simulink model "meat_1024pt_lwip_led"  (Simulink 6.2)
settings: Solver=ode45  StartTime=0.0  StopTime=20000  RelTol=1e-3
undefined symbols (not defined in the file): bit_rev, iBOB, pfb_coeff_gen_calc
libraries: xbsIndex_r3 x1078, casper_library x97, xps_library x30
(part 8 of 8)

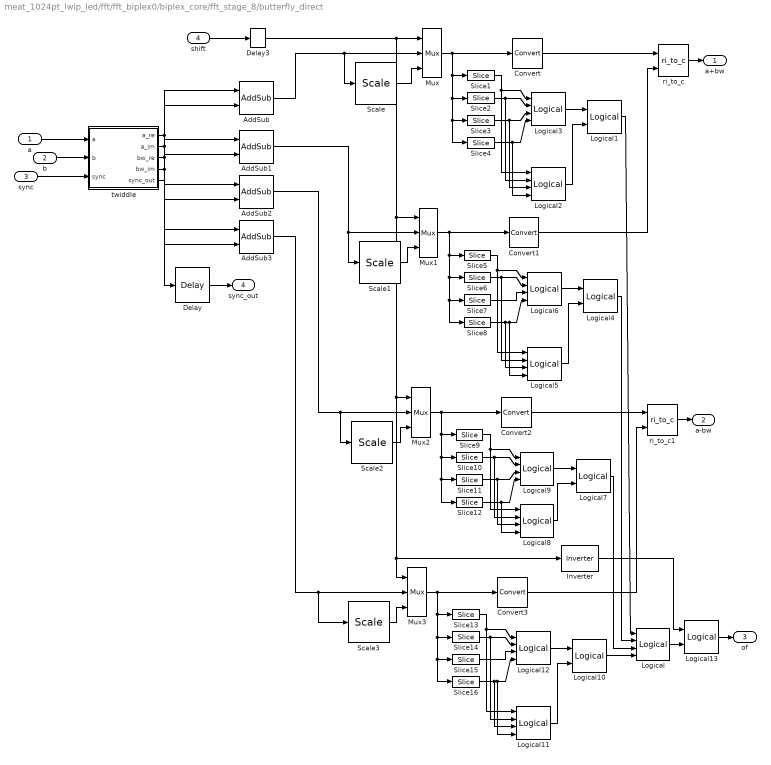
== system meat_1024pt_lwip_led/fft/fft_biplex0/biplex_core/fft_stage_8/butterfly_direct ==
  a : Inport  Port=1  LatchInput=off
  b : Inport  Port=2  LatchInput=off
  sync : Inport  Port=3  LatchInput=off
  shift : Inport  Port=4  LatchInput=off
  AddSub : xbsIndex_r3/AddSub  mode=Addition  precision=Full  arith_type=Unsigned  n_bits=8  bin_pt=2  quantization=Truncate  overflow=Wrap  latency=add_latency  explicit_period=off  period=1  use_carryin=off  use_carryout=off  en=off  dbl_ovrd=off  show_param=on  use_core=on  pipeline=on  use_rpm=on  gen_core=on
      settings: xl_area=[0, 0, 0, 0, 0, 0, 0]
  AddSub1 : xbsIndex_r3/AddSub  mode=Addition  precision=Full  arith_type=Unsigned  n_bits=8  bin_pt=2  quantization=Truncate  overflow=Wrap  latency=add_latency  explicit_period=off  period=1  use_carryin=off  use_carryout=off  en=off  dbl_ovrd=off  show_param=on  use_core=on  pipeline=on  use_rpm=on  gen_core=on
      settings: xl_area=[0, 0, 0, 0, 0, 0, 0]
  AddSub2 : xbsIndex_r3/AddSub  mode=Subtraction  precision=Full  arith_type=Unsigned  n_bits=8  bin_pt=2  quantization=Truncate  overflow=Wrap  latency=add_latency  explicit_period=off  period=1  use_carryin=off  use_carryout=off  en=off  dbl_ovrd=off  show_param=on  use_core=on  pipeline=on  use_rpm=on  gen_core=on
      settings: xl_area=[0, 0, 0, 0, 0, 0, 0]
  AddSub3 : xbsIndex_r3/AddSub  mode=Subtraction  precision=Full  arith_type=Unsigned  n_bits=8  bin_pt=2  quantization=Truncate  overflow=Wrap  latency=add_latency  explicit_period=off  period=1  use_carryin=off  use_carryout=off  en=off  dbl_ovrd=off  show_param=on  use_core=on  pipeline=on  use_rpm=on  gen_core=on
      settings: xl_area=[0, 0, 0, 0, 0, 0, 0]
  Convert{,1..3} (4 alike) : xbsIndex_r3/Convert  arith_type="Signed  (2's comp)"  n_bits=BitWidth  bin_pt=BitWidth-1  quantization=Truncate  overflow=Wrap  latency=add_latency  explicit_period=off  period=1  dbl_ovrd=off  show_param=off  inserted_by_tool=off  pipeline=off
      settings: xl_area=[0, 0, 0, 0, 0, 0, 0]
  Delay : xbsIndex_r3/Delay  latency=2 * add_latency + 1  reg_retiming=off  explicit_period=off  period=1  en=off  accept_only_valid=off  init_zero=on  dbl_ovrd=off  show_param=off
      settings: xl_area=[0, 0, 0, 0, 0, 0, 0]
  Delay3 : xbsIndex_r3/Delay  latency=1  reg_retiming=off  explicit_period=off  period=1  en=off  accept_only_valid=off  init_zero=on  dbl_ovrd=off  show_param=off
      settings: xl_area=[0, 0, 0, 0, 0, 0, 0]
  Inverter : xbsIndex_r3/Inverter  latency=0  explicit_period=off  period=1  en=off  dbl_ovrd=off  show_param=off
      settings: xl_area=[0, 0, 0, 0, 0, 0, 0]
  Logical : xbsIndex_r3/Logical  logical_function=OR  inputs=4  precision=Full  arith_type=Unsigned  n_bits=8  bin_pt=2  align_bp=on  latency=1  explicit_period=off  period=1  en=off  dbl_ovrd=off  show_param=off
      settings: xl_area=[0, 0, 0, 0, 0, 0, 0]
  Logical{1,4,7,10} (4 alike) : xbsIndex_r3/Logical  logical_function=OR  inputs=2  precision=Full  arith_type=Unsigned  n_bits=8  bin_pt=2  align_bp=off  latency=1  explicit_period=off  period=1  en=off  dbl_ovrd=off  show_param=off
      settings: xl_area=[0, 0, 0, 0, 0, 0, 0]
  Logical{2,5,8,11} (4 alike) : xbsIndex_r3/Logical  logical_function=NOR  inputs=4  precision=Full  arith_type=Unsigned  n_bits=8  bin_pt=2  align_bp=off  latency=1  explicit_period=off  period=1  en=off  dbl_ovrd=off  show_param=off
      settings: xl_area=[0, 0, 0, 0, 0, 0, 0]
  Logical{3,6,9,12} (4 alike) : xbsIndex_r3/Logical  logical_function=AND  inputs=4  precision=Full  arith_type=Unsigned  n_bits=8  bin_pt=2  align_bp=off  latency=1  explicit_period=off  period=1  en=off  dbl_ovrd=off  show_param=off
      settings: xl_area=[0, 0, 0, 0, 0, 0, 0]
  Logical13 : xbsIndex_r3/Logical  logical_function=AND  inputs=2  precision=Full  arith_type=Unsigned  n_bits=8  bin_pt=2  align_bp=off  latency=1  explicit_period=off  period=1  en=off  dbl_ovrd=off  show_param=off
      settings: xl_area=[0, 0, 0, 0, 0, 0, 0]
  Mux{,1..3} (4 alike) : xbsIndex_r3/Mux  inputs=2  precision=Full  arith_type="Signed  (2's comp)"  n_bits=8  bin_pt=2  quantization=Truncate  overflow=Wrap  latency=1  explicit_period=off  period=1  en=off  dbl_ovrd=off  show_param=off  mux_type=off  use_rpm=off  gen_core=off
      settings: xl_area=[0, 0, 0, 0, 0, 0, 0]
  Scale{,1..3} (4 alike) : xbsIndex_r3/Scale  scale_factor=-1  explicit_period=off  period=1  dbl_ovrd=off
  Slice{1,5,9,13} (4 alike) : xbsIndex_r3/Slice  mode=Upper Bit Location + Width  nbits=1  bit1=0  base1=MSB of Input  bit0=0  base0=LSB of Input  boolean_output=on  explicit_period=off  period=1  dbl_ovrd=off
  Slice{2,6,10,14} (4 alike) : xbsIndex_r3/Slice  mode=Upper Bit Location + Width  nbits=1  bit1=-1  base1=MSB of Input  bit0=0  base0=LSB of Input  boolean_output=on  explicit_period=off  period=1  dbl_ovrd=off
  Slice{3,7,11,15} (4 alike) : xbsIndex_r3/Slice  mode=Upper Bit Location + Width  nbits=1  bit1=-2  base1=MSB of Input  bit0=0  base0=LSB of Input  boolean_output=on  explicit_period=off  period=1  dbl_ovrd=off
  Slice{4,8,12,16} (4 alike) : xbsIndex_r3/Slice  mode=Upper Bit Location + Width  nbits=1  bit1=-3  base1=MSB of Input  bit0=0  base0=LSB of Input  boolean_output=on  explicit_period=off  period=1  dbl_ovrd=off
  ri_to_c : casper_library/Misc/ri_to_c
  ri_to_c1 : casper_library/Misc/ri_to_c
  twiddle : Subsystem  BlockChoice=twiddle_general_3mult
      link override twiddle_general_3mult: Coeffs=[exp(-2*pi*1j*(bit_rev(Coeffs, FFTSize-1))/2^FFTSize)]  StepPeriod=2  BitWidth=18  add_latency=3  mult_latency=4  bram_latency=3
      link override twiddle_general_3mult/coeff_gen: BlockChoice=br_coeff_gen
      link override twiddle_general_3mult/coeff_gen/br_coeff_gen: Coeffs=[1 2 3 4 5 6 7]  StepPeriod=4  BitWidth=10  bram_latency=6
      link override twiddle_general_3mult/coeff_gen/br_coeff_gen/ROM: distributed_mem=off
      link override twiddle_general_3mult/coeff_gen/br_coeff_gen/ROM1: distributed_mem=off
      link override twiddle_general_3mult/coeff_gen/static_coeff_gen/Constant: equ=P=C
      link override twiddle_general_3mult/coeff_gen/static_coeff_gen/Constant1: equ=P=C
      settings: AttributesFormatString=%<BlockChoice>  TemplateBlock=casper_library/FFTs/Twiddle/twiddle  MemberBlocks=twiddle_coeff_0,twiddle_coeff_1,twiddle_general_3mult,twiddle_general_4mult,twiddle_stage_2
  a+bw : Outport
  a-bw : Outport  Port=2
  of : Outport  Port=3
  sync_out : Outport  Port=4
  wires:
  Inverter/1 -> Logical13/1
  Logical13/1 -> of/1
  Logical/1 -> Logical13/2
  Delay3/1 -> Inverter/1, Mux3/1, Mux2/1, Mux1/1, Mux/1
  Logical7/1 -> Logical/3
  AddSub3/1 -> Scale3/1, Mux3/2
  Logical10/1 -> Logical/4
  Logical11/1 -> Logical10/2
  Logical12/1 -> Logical10/1
  Slice16/1 -> Logical11/3, Logical11/4, Logical12/4
  Slice15/1 -> Logical12/3
  Slice14/1 -> Logical11/2, Logical12/2
  Slice13/1 -> Logical11/1, Logical12/1
  Convert3/1 -> ri_to_c1/2
  Scale3/1 -> Mux3/3
  Mux3/1 -> Slice16/1, Slice15/1, Slice14/1, Slice13/1, Convert3/1
  AddSub2/1 -> Scale2/1, Mux2/2
  Logical8/1 -> Logical7/2
  Logical9/1 -> Logical7/1
  Slice12/1 -> Logical8/4, Logical9/4
  Slice11/1 -> Logical8/3, Logical9/3
  Slice10/1 -> Logical8/2, Logical9/2
  Slice9/1 -> Logical8/1, Logical9/1
  Convert2/1 -> ri_to_c1/1
  Scale2/1 -> Mux2/3
  Mux2/1 -> Slice12/1, Slice11/1, Slice10/1, Slice9/1, Convert2/1
  Logical4/1 -> Logical/2
  Logical5/1 -> Logical4/2
  Logical6/1 -> Logical4/1
  Slice8/1 -> Logical5/3, Logical5/4, Logical6/4
  Slice7/1 -> Logical6/3
  Slice6/1 -> Logical5/2, Logical6/2
  Slice5/1 -> Logical5/1, Logical6/1
  Convert1/1 -> ri_to_c/2
  Scale1/1 -> Mux1/3
  Mux1/1 -> Slice8/1, Slice7/1, Slice6/1, Slice5/1, Convert1/1
  Logical1/1 -> Logical/1
  Logical2/1 -> Logical1/2
  Logical3/1 -> Logical1/1
  Slice4/1 -> Logical2/4, Logical3/4
  Slice3/1 -> Logical2/3, Logical3/3
  Slice2/1 -> Logical2/2, Logical3/2
  Slice1/1 -> Logical2/1, Logical3/1
  Convert/1 -> ri_to_c/1
  Scale/1 -> Mux/3
  Mux/1 -> Slice4/1, Slice3/1, Slice2/1, Slice1/1, Convert/1
  shift/1 -> Delay3/1
  AddSub1/1 -> Scale1/1, Mux1/2
  AddSub/1 -> Scale/1, Mux/2
  Delay/1 -> sync_out/1
  ri_to_c1/1 -> a-bw/1
  ri_to_c/1 -> a+bw/1
  a/1 -> twiddle/1(a)
  b/1 -> twiddle/2(b)
  sync/1 -> twiddle/3(sync)
  twiddle/1(a_re) -> AddSub/1, AddSub2/1
  twiddle/2(a_im) -> AddSub1/1, AddSub3/1
  twiddle/3(bw_re) -> AddSub/2, AddSub2/2
  twiddle/4(bw_im) -> AddSub1/2, AddSub3/2
  twiddle/5(sync_out) -> Delay/1

== system meat_1024pt_lwip_led/fft/fft_biplex0/biplex_core/fft_stage_8/delay_b ==
  In1 : Inport  Port=1  LatchInput=off
  delay_slr : casper_library/Delays/delay_slr  DelayLen=2^(FFTSize-FFTStage)
  Out1 : Outport
  wires:
  In1/1 -> delay_slr/1
  delay_slr/1 -> Out1/1

== system meat_1024pt_lwip_led/fft/fft_biplex0/biplex_core/fft_stage_8/delay_f ==
  In1 : Inport  Port=1  LatchInput=off
  delay_slr : casper_library/Delays/delay_slr  DelayLen=2^(FFTSize-FFTStage)
  Out1 : Outport
  wires:
  In1/1 -> delay_slr/1
  delay_slr/1 -> Out1/1

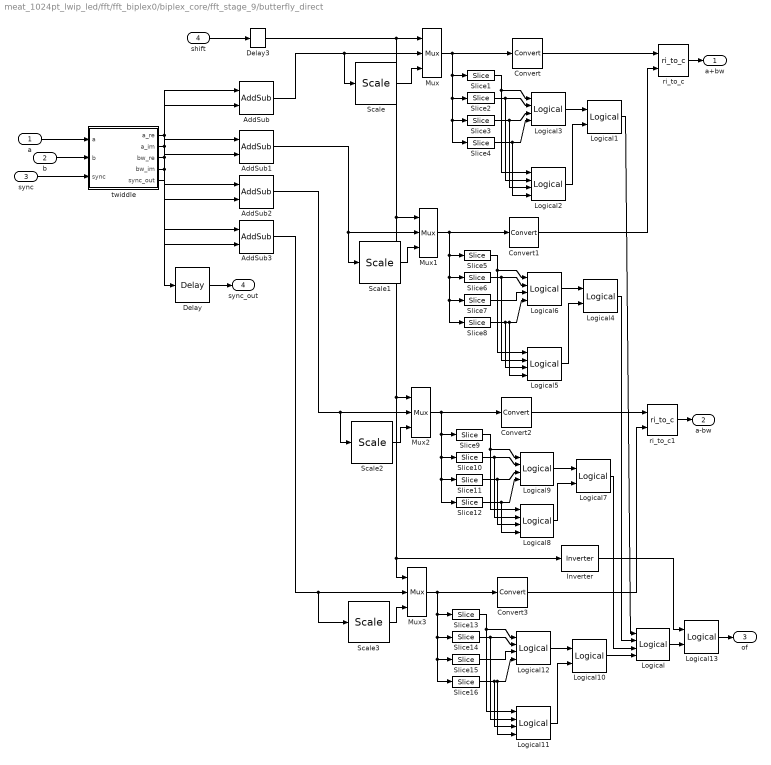
== system meat_1024pt_lwip_led/fft/fft_biplex0/biplex_core/fft_stage_9/butterfly_direct ==
  a : Inport  Port=1  LatchInput=off
  b : Inport  Port=2  LatchInput=off
  sync : Inport  Port=3  LatchInput=off
  shift : Inport  Port=4  LatchInput=off
  AddSub : xbsIndex_r3/AddSub  mode=Addition  precision=Full  arith_type=Unsigned  n_bits=8  bin_pt=2  quantization=Truncate  overflow=Wrap  latency=add_latency  explicit_period=off  period=1  use_carryin=off  use_carryout=off  en=off  dbl_ovrd=off  show_param=on  use_core=on  pipeline=on  use_rpm=on  gen_core=on
      settings: xl_area=[0, 0, 0, 0, 0, 0, 0]
  AddSub1 : xbsIndex_r3/AddSub  mode=Addition  precision=Full  arith_type=Unsigned  n_bits=8  bin_pt=2  quantization=Truncate  overflow=Wrap  latency=add_latency  explicit_period=off  period=1  use_carryin=off  use_carryout=off  en=off  dbl_ovrd=off  show_param=on  use_core=on  pipeline=on  use_rpm=on  gen_core=on
      settings: xl_area=[0, 0, 0, 0, 0, 0, 0]
  AddSub2 : xbsIndex_r3/AddSub  mode=Subtraction  precision=Full  arith_type=Unsigned  n_bits=8  bin_pt=2  quantization=Truncate  overflow=Wrap  latency=add_latency  explicit_period=off  period=1  use_carryin=off  use_carryout=off  en=off  dbl_ovrd=off  show_param=on  use_core=on  pipeline=on  use_rpm=on  gen_core=on
      settings: xl_area=[0, 0, 0, 0, 0, 0, 0]
  AddSub3 : xbsIndex_r3/AddSub  mode=Subtraction  precision=Full  arith_type=Unsigned  n_bits=8  bin_pt=2  quantization=Truncate  overflow=Wrap  latency=add_latency  explicit_period=off  period=1  use_carryin=off  use_carryout=off  en=off  dbl_ovrd=off  show_param=on  use_core=on  pipeline=on  use_rpm=on  gen_core=on
      settings: xl_area=[0, 0, 0, 0, 0, 0, 0]
  Convert{,1..3} (4 alike) : xbsIndex_r3/Convert  arith_type="Signed  (2's comp)"  n_bits=BitWidth  bin_pt=BitWidth-1  quantization=Truncate  overflow=Wrap  latency=add_latency  explicit_period=off  period=1  dbl_ovrd=off  show_param=off  inserted_by_tool=off  pipeline=off
      settings: xl_area=[0, 0, 0, 0, 0, 0, 0]
  Delay : xbsIndex_r3/Delay  latency=2 * add_latency + 1  reg_retiming=off  explicit_period=off  period=1  en=off  accept_only_valid=off  init_zero=on  dbl_ovrd=off  show_param=off
      settings: xl_area=[0, 0, 0, 0, 0, 0, 0]
  Delay3 : xbsIndex_r3/Delay  latency=1  reg_retiming=off  explicit_period=off  period=1  en=off  accept_only_valid=off  init_zero=on  dbl_ovrd=off  show_param=off
      settings: xl_area=[0, 0, 0, 0, 0, 0, 0]
  Inverter : xbsIndex_r3/Inverter  latency=0  explicit_period=off  period=1  en=off  dbl_ovrd=off  show_param=off
      settings: xl_area=[0, 0, 0, 0, 0, 0, 0]
  Logical : xbsIndex_r3/Logical  logical_function=OR  inputs=4  precision=Full  arith_type=Unsigned  n_bits=8  bin_pt=2  align_bp=on  latency=1  explicit_period=off  period=1  en=off  dbl_ovrd=off  show_param=off
      settings: xl_area=[0, 0, 0, 0, 0, 0, 0]
  Logical{1,4,7,10} (4 alike) : xbsIndex_r3/Logical  logical_function=OR  inputs=2  precision=Full  arith_type=Unsigned  n_bits=8  bin_pt=2  align_bp=off  latency=1  explicit_period=off  period=1  en=off  dbl_ovrd=off  show_param=off
      settings: xl_area=[0, 0, 0, 0, 0, 0, 0]
  Logical{2,5,8,11} (4 alike) : xbsIndex_r3/Logical  logical_function=NOR  inputs=4  precision=Full  arith_type=Unsigned  n_bits=8  bin_pt=2  align_bp=off  latency=1  explicit_period=off  period=1  en=off  dbl_ovrd=off  show_param=off
      settings: xl_area=[0, 0, 0, 0, 0, 0, 0]
  Logical{3,6,9,12} (4 alike) : xbsIndex_r3/Logical  logical_function=AND  inputs=4  precision=Full  arith_type=Unsigned  n_bits=8  bin_pt=2  align_bp=off  latency=1  explicit_period=off  period=1  en=off  dbl_ovrd=off  show_param=off
      settings: xl_area=[0, 0, 0, 0, 0, 0, 0]
  Logical13 : xbsIndex_r3/Logical  logical_function=AND  inputs=2  precision=Full  arith_type=Unsigned  n_bits=8  bin_pt=2  align_bp=off  latency=1  explicit_period=off  period=1  en=off  dbl_ovrd=off  show_param=off
      settings: xl_area=[0, 0, 0, 0, 0, 0, 0]
  Mux{,1..3} (4 alike) : xbsIndex_r3/Mux  inputs=2  precision=Full  arith_type="Signed  (2's comp)"  n_bits=8  bin_pt=2  quantization=Truncate  overflow=Wrap  latency=1  explicit_period=off  period=1  en=off  dbl_ovrd=off  show_param=off  mux_type=off  use_rpm=off  gen_core=off
      settings: xl_area=[0, 0, 0, 0, 0, 0, 0]
  Scale{,1..3} (4 alike) : xbsIndex_r3/Scale  scale_factor=-1  explicit_period=off  period=1  dbl_ovrd=off
  Slice{1,5,9,13} (4 alike) : xbsIndex_r3/Slice  mode=Upper Bit Location + Width  nbits=1  bit1=0  base1=MSB of Input  bit0=0  base0=LSB of Input  boolean_output=on  explicit_period=off  period=1  dbl_ovrd=off
  Slice{2,6,10,14} (4 alike) : xbsIndex_r3/Slice  mode=Upper Bit Location + Width  nbits=1  bit1=-1  base1=MSB of Input  bit0=0  base0=LSB of Input  boolean_output=on  explicit_period=off  period=1  dbl_ovrd=off
  Slice{3,7,11,15} (4 alike) : xbsIndex_r3/Slice  mode=Upper Bit Location + Width  nbits=1  bit1=-2  base1=MSB of Input  bit0=0  base0=LSB of Input  boolean_output=on  explicit_period=off  period=1  dbl_ovrd=off
  Slice{4,8,12,16} (4 alike) : xbsIndex_r3/Slice  mode=Upper Bit Location + Width  nbits=1  bit1=-3  base1=MSB of Input  bit0=0  base0=LSB of Input  boolean_output=on  explicit_period=off  period=1  dbl_ovrd=off
  ri_to_c : casper_library/Misc/ri_to_c
  ri_to_c1 : casper_library/Misc/ri_to_c
  twiddle : Subsystem  BlockChoice=twiddle_general_3mult
      link override twiddle_general_3mult: Coeffs=[exp(-2*pi*1j*(bit_rev(Coeffs, FFTSize-1))/2^FFTSize)]  StepPeriod=1  BitWidth=18  add_latency=3  mult_latency=4  bram_latency=3
      link override twiddle_general_3mult/coeff_gen: BlockChoice=br_coeff_gen
      link override twiddle_general_3mult/coeff_gen/br_coeff_gen: Coeffs=[1 2 3 4 5 6 7]  StepPeriod=4  BitWidth=10  bram_latency=6
      link override twiddle_general_3mult/coeff_gen/br_coeff_gen/ROM: distributed_mem=off
      link override twiddle_general_3mult/coeff_gen/br_coeff_gen/ROM1: distributed_mem=off
      link override twiddle_general_3mult/coeff_gen/static_coeff_gen/Constant: equ=P=C
      link override twiddle_general_3mult/coeff_gen/static_coeff_gen/Constant1: equ=P=C
      settings: AttributesFormatString=%<BlockChoice>  TemplateBlock=casper_library/FFTs/Twiddle/twiddle  MemberBlocks=twiddle_coeff_0,twiddle_coeff_1,twiddle_general_3mult,twiddle_general_4mult,twiddle_stage_2
  a+bw : Outport
  a-bw : Outport  Port=2
  of : Outport  Port=3
  sync_out : Outport  Port=4
  wires:
  Inverter/1 -> Logical13/1
  Logical13/1 -> of/1
  Logical/1 -> Logical13/2
  Delay3/1 -> Inverter/1, Mux3/1, Mux2/1, Mux1/1, Mux/1
  Logical7/1 -> Logical/3
  AddSub3/1 -> Scale3/1, Mux3/2
  Logical10/1 -> Logical/4
  Logical11/1 -> Logical10/2
  Logical12/1 -> Logical10/1
  Slice16/1 -> Logical11/3, Logical11/4, Logical12/4
  Slice15/1 -> Logical12/3
  Slice14/1 -> Logical11/2, Logical12/2
  Slice13/1 -> Logical11/1, Logical12/1
  Convert3/1 -> ri_to_c1/2
  Scale3/1 -> Mux3/3
  Mux3/1 -> Slice16/1, Slice15/1, Slice14/1, Slice13/1, Convert3/1
  AddSub2/1 -> Scale2/1, Mux2/2
  Logical8/1 -> Logical7/2
  Logical9/1 -> Logical7/1
  Slice12/1 -> Logical8/4, Logical9/4
  Slice11/1 -> Logical8/3, Logical9/3
  Slice10/1 -> Logical8/2, Logical9/2
  Slice9/1 -> Logical8/1, Logical9/1
  Convert2/1 -> ri_to_c1/1
  Scale2/1 -> Mux2/3
  Mux2/1 -> Slice12/1, Slice11/1, Slice10/1, Slice9/1, Convert2/1
  Logical4/1 -> Logical/2
  Logical5/1 -> Logical4/2
  Logical6/1 -> Logical4/1
  Slice8/1 -> Logical5/3, Logical5/4, Logical6/4
  Slice7/1 -> Logical6/3
  Slice6/1 -> Logical5/2, Logical6/2
  Slice5/1 -> Logical5/1, Logical6/1
  Convert1/1 -> ri_to_c/2
  Scale1/1 -> Mux1/3
  Mux1/1 -> Slice8/1, Slice7/1, Slice6/1, Slice5/1, Convert1/1
  Logical1/1 -> Logical/1
  Logical2/1 -> Logical1/2
  Logical3/1 -> Logical1/1
  Slice4/1 -> Logical2/4, Logical3/4
  Slice3/1 -> Logical2/3, Logical3/3
  Slice2/1 -> Logical2/2, Logical3/2
  Slice1/1 -> Logical2/1, Logical3/1
  Convert/1 -> ri_to_c/1
  Scale/1 -> Mux/3
  Mux/1 -> Slice4/1, Slice3/1, Slice2/1, Slice1/1, Convert/1
  shift/1 -> Delay3/1
  AddSub1/1 -> Scale1/1, Mux1/2
  AddSub/1 -> Scale/1, Mux/2
  Delay/1 -> sync_out/1
  ri_to_c1/1 -> a-bw/1
  ri_to_c/1 -> a+bw/1
  a/1 -> twiddle/1(a)
  b/1 -> twiddle/2(b)
  sync/1 -> twiddle/3(sync)
  twiddle/1(a_re) -> AddSub/1, AddSub2/1
  twiddle/2(a_im) -> AddSub1/1, AddSub3/1
  twiddle/3(bw_re) -> AddSub/2, AddSub2/2
  twiddle/4(bw_im) -> AddSub1/2, AddSub3/2
  twiddle/5(sync_out) -> Delay/1

== system meat_1024pt_lwip_led/fft/fft_biplex0/biplex_core/fft_stage_9/delay_b ==
  In1 : Inport  Port=1  LatchInput=off
  delay_slr : casper_library/Delays/delay_slr  DelayLen=2^(FFTSize-FFTStage)
  Out1 : Outport
  wires:
  In1/1 -> delay_slr/1
  delay_slr/1 -> Out1/1

== system meat_1024pt_lwip_led/fft/fft_biplex0/biplex_core/fft_stage_9/delay_f ==
  In1 : Inport  Port=1  LatchInput=off
  delay_slr : casper_library/Delays/delay_slr  DelayLen=2^(FFTSize-FFTStage)
  Out1 : Outport
  wires:
  In1/1 -> delay_slr/1
  delay_slr/1 -> Out1/1

== system meat_1024pt_lwip_led/fft/fft_biplex0/biplex_cplx_unscrambler/reorder/map1 ==
  din : Inport  Port=1  LatchInput=off
  Concat : xbsIndex_r3/Concat  num_inputs=10  explicit_period=off  period=1  dbl_ovrd=off
  Uncram : Subsystem  AncestorBlock=casper_library/Misc/uncram  mask(uncram){num_slice=10, slice_width=1, bin_pt=0, arith_type=0}
      mask prompts: num_slice "Number of slices"; slice_width "Slice Width"; bin_pt "Output Binary Point"; arith_type "Output Arithmetic Type (0=Unsigned, 1=Signed)"
      mask help: Takes a concatenated input and slices it up into even pieces and reinterprets them as signed fixed point numbers with a given binary point.
      mask init:
      | uncram_init(gcb, ...
      |     'num_slice', num_slice, ...
      |     'slice_width', slice_width, ...
      |     'bin_pt', bin_pt, ...
      |     'arith_type', arith_type);
      settings: AttributesFormatString=UFix_1_0
  expr0 : xbsIndex_r3/Expression  expression=(in08)|(in00&~in00)|(in01&~in01)|(in02&~in02)|(in03&~in03)|(in04&~in04)|(in05&~in05)|(in06&~in06)|(in07&~in07)|(in08&~in08)|(in09&~in09)  precision=Full  arith_type=Unsigned  n_bits=8  bin_pt=2  align_bp=on  latency=0  explicit_period=off  period=1  en=off  dbl_ovrd=off  show_param=off
      settings: xl_area=[0, 0, 0, 0, 0, 0, 0]
  expr1 : xbsIndex_r3/Expression  expression=(in07)|(in00&~in00)|(in01&~in01)|(in02&~in02)|(in03&~in03)|(in04&~in04)|(in05&~in05)|(in06&~in06)|(in07&~in07)|(in08&~in08)|(in09&~in09)  precision=Full  arith_type=Unsigned  n_bits=8  bin_pt=2  align_bp=on  latency=0  explicit_period=off  period=1  en=off  dbl_ovrd=off  show_param=off
      settings: xl_area=[0, 0, 0, 0, 0, 0, 0]
  expr2 : xbsIndex_r3/Expression  expression=(in06)|(in00&~in00)|(in01&~in01)|(in02&~in02)|(in03&~in03)|(in04&~in04)|(in05&~in05)|(in06&~in06)|(in07&~in07)|(in08&~in08)|(in09&~in09)  precision=Full  arith_type=Unsigned  n_bits=8  bin_pt=2  align_bp=on  latency=0  explicit_period=off  period=1  en=off  dbl_ovrd=off  show_param=off
      settings: xl_area=[0, 0, 0, 0, 0, 0, 0]
  expr3 : xbsIndex_r3/Expression  expression=(in05)|(in00&~in00)|(in01&~in01)|(in02&~in02)|(in03&~in03)|(in04&~in04)|(in05&~in05)|(in06&~in06)|(in07&~in07)|(in08&~in08)|(in09&~in09)  precision=Full  arith_type=Unsigned  n_bits=8  bin_pt=2  align_bp=on  latency=0  explicit_period=off  period=1  en=off  dbl_ovrd=off  show_param=off
      settings: xl_area=[0, 0, 0, 0, 0, 0, 0]
  expr4 : xbsIndex_r3/Expression  expression=(in04)|(in00&~in00)|(in01&~in01)|(in02&~in02)|(in03&~in03)|(in04&~in04)|(in05&~in05)|(in06&~in06)|(in07&~in07)|(in08&~in08)|(in09&~in09)  precision=Full  arith_type=Unsigned  n_bits=8  bin_pt=2  align_bp=on  latency=0  explicit_period=off  period=1  en=off  dbl_ovrd=off  show_param=off
      settings: xl_area=[0, 0, 0, 0, 0, 0, 0]
  expr5 : xbsIndex_r3/Expression  expression=(in03)|(in00&~in00)|(in01&~in01)|(in02&~in02)|(in03&~in03)|(in04&~in04)|(in05&~in05)|(in06&~in06)|(in07&~in07)|(in08&~in08)|(in09&~in09)  precision=Full  arith_type=Unsigned  n_bits=8  bin_pt=2  align_bp=on  latency=0  explicit_period=off  period=1  en=off  dbl_ovrd=off  show_param=off
      settings: xl_area=[0, 0, 0, 0, 0, 0, 0]
  expr6 : xbsIndex_r3/Expression  expression=(in02)|(in00&~in00)|(in01&~in01)|(in02&~in02)|(in03&~in03)|(in04&~in04)|(in05&~in05)|(in06&~in06)|(in07&~in07)|(in08&~in08)|(in09&~in09)  precision=Full  arith_type=Unsigned  n_bits=8  bin_pt=2  align_bp=on  latency=0  explicit_period=off  period=1  en=off  dbl_ovrd=off  show_param=off
      settings: xl_area=[0, 0, 0, 0, 0, 0, 0]
  expr7 : xbsIndex_r3/Expression  expression=(in01)|(in00&~in00)|(in01&~in01)|(in02&~in02)|(in03&~in03)|(in04&~in04)|(in05&~in05)|(in06&~in06)|(in07&~in07)|(in08&~in08)|(in09&~in09)  precision=Full  arith_type=Unsigned  n_bits=8  bin_pt=2  align_bp=on  latency=0  explicit_period=off  period=1  en=off  dbl_ovrd=off  show_param=off
      settings: xl_area=[0, 0, 0, 0, 0, 0, 0]
  expr8 : xbsIndex_r3/Expression  expression=(in00)|(in00&~in00)|(in01&~in01)|(in02&~in02)|(in03&~in03)|(in04&~in04)|(in05&~in05)|(in06&~in06)|(in07&~in07)|(in08&~in08)|(in09&~in09)  precision=Full  arith_type=Unsigned  n_bits=8  bin_pt=2  align_bp=on  latency=0  explicit_period=off  period=1  en=off  dbl_ovrd=off  show_param=off
      settings: xl_area=[0, 0, 0, 0, 0, 0, 0]
  expr9 : xbsIndex_r3/Expression  expression=(in09)|(in00&~in00)|(in01&~in01)|(in02&~in02)|(in03&~in03)|(in04&~in04)|(in05&~in05)|(in06&~in06)|(in07&~in07)|(in08&~in08)|(in09&~in09)  precision=Full  arith_type=Unsigned  n_bits=8  bin_pt=2  align_bp=on  latency=0  explicit_period=off  period=1  en=off  dbl_ovrd=off  show_param=off
      settings: xl_area=[0, 0, 0, 0, 0, 0, 0]
  dout : Outport
  wires:
  Uncram/10(Out10) -> expr0/1, expr1/1, expr2/1, expr3/1, expr4/1, expr5/1, expr6/1, expr7/1, expr8/1, expr9/1
  Uncram/9(Out9) -> expr0/2, expr1/2, expr2/2, expr3/2, expr4/2, expr5/2, expr6/2, expr7/2, expr8/2, expr9/2
  Uncram/8(Out8) -> expr0/3, expr1/3, expr2/3, expr3/3, expr4/3, expr5/3, expr6/3, expr7/3, expr8/3, expr9/3
  Uncram/7(Out7) -> expr0/4, expr1/4, expr2/4, expr3/4, expr4/4, expr5/4, expr6/4, expr7/4, expr8/4, expr9/4
  Uncram/6(Out6) -> expr0/5, expr1/5, expr2/5, expr3/5, expr4/5, expr5/5, expr6/5, expr7/5, expr8/5, expr9/5
  Uncram/5(Out5) -> expr0/6, expr1/6, expr2/6, expr3/6, expr4/6, expr5/6, expr6/6, expr7/6, expr8/6, expr9/6
  Uncram/4(Out4) -> expr0/7, expr1/7, expr2/7, expr3/7, expr4/7, expr5/7, expr6/7, expr7/7, expr8/7, expr9/7
  Uncram/3(Out3) -> expr0/8, expr1/8, expr2/8, expr3/8, expr4/8, expr5/8, expr6/8, expr7/8, expr8/8, expr9/8
  Uncram/2(Out2) -> expr0/9, expr1/9, expr2/9, expr3/9, expr4/9, expr5/9, expr6/9, expr7/9, expr8/9, expr9/9
  Uncram/1(Out1) -> expr0/10, expr1/10, expr2/10, expr3/10, expr4/10, expr5/10, expr6/10, expr7/10, expr8/10, expr9/10
  expr0/1 -> Concat/10
  expr1/1 -> Concat/9
  expr2/1 -> Concat/8
  expr3/1 -> Concat/7
  expr4/1 -> Concat/6
  expr5/1 -> Concat/5
  expr6/1 -> Concat/4
  expr7/1 -> Concat/3
  expr8/1 -> Concat/2
  expr9/1 -> Concat/1
  din/1 -> Uncram/1(In)
  Concat/1 -> dout/1

== system meat_1024pt_lwip_led/fft/fft_biplex0/biplex_cplx_unscrambler/reorder1/map1 ==
  din : Inport  Port=1  LatchInput=off
  Concat : xbsIndex_r3/Concat  num_inputs=10  explicit_period=off  period=1  dbl_ovrd=off
  Uncram : Subsystem  AncestorBlock=casper_library/Misc/uncram  mask(uncram){num_slice=10, slice_width=1, bin_pt=0, arith_type=0}
      mask prompts: num_slice "Number of slices"; slice_width "Slice Width"; bin_pt "Output Binary Point"; arith_type "Output Arithmetic Type (0=Unsigned, 1=Signed)"
      mask help: Takes a concatenated input and slices it up into even pieces and reinterprets them as signed fixed point numbers with a given binary point.
      mask init:
      | uncram_init(gcb, ...
      |     'num_slice', num_slice, ...
      |     'slice_width', slice_width, ...
      |     'bin_pt', bin_pt, ...
      |     'arith_type', arith_type);
      settings: AttributesFormatString=UFix_1_0
  expr0 : xbsIndex_r3/Expression  expression=(in08)|(in00&~in00)|(in01&~in01)|(in02&~in02)|(in03&~in03)|(in04&~in04)|(in05&~in05)|(in06&~in06)|(in07&~in07)|(in08&~in08)|(in09&~in09)  precision=Full  arith_type=Unsigned  n_bits=8  bin_pt=2  align_bp=on  latency=0  explicit_period=off  period=1  en=off  dbl_ovrd=off  show_param=off
      settings: xl_area=[0, 0, 0, 0, 0, 0, 0]
  expr1 : xbsIndex_r3/Expression  expression=(in07)|(in00&~in00)|(in01&~in01)|(in02&~in02)|(in03&~in03)|(in04&~in04)|(in05&~in05)|(in06&~in06)|(in07&~in07)|(in08&~in08)|(in09&~in09)  precision=Full  arith_type=Unsigned  n_bits=8  bin_pt=2  align_bp=on  latency=0  explicit_period=off  period=1  en=off  dbl_ovrd=off  show_param=off
      settings: xl_area=[0, 0, 0, 0, 0, 0, 0]
  expr2 : xbsIndex_r3/Expression  expression=(in06)|(in00&~in00)|(in01&~in01)|(in02&~in02)|(in03&~in03)|(in04&~in04)|(in05&~in05)|(in06&~in06)|(in07&~in07)|(in08&~in08)|(in09&~in09)  precision=Full  arith_type=Unsigned  n_bits=8  bin_pt=2  align_bp=on  latency=0  explicit_period=off  period=1  en=off  dbl_ovrd=off  show_param=off
      settings: xl_area=[0, 0, 0, 0, 0, 0, 0]
  expr3 : xbsIndex_r3/Expression  expression=(in05)|(in00&~in00)|(in01&~in01)|(in02&~in02)|(in03&~in03)|(in04&~in04)|(in05&~in05)|(in06&~in06)|(in07&~in07)|(in08&~in08)|(in09&~in09)  precision=Full  arith_type=Unsigned  n_bits=8  bin_pt=2  align_bp=on  latency=0  explicit_period=off  period=1  en=off  dbl_ovrd=off  show_param=off
      settings: xl_area=[0, 0, 0, 0, 0, 0, 0]
  expr4 : xbsIndex_r3/Expression  expression=(in04)|(in00&~in00)|(in01&~in01)|(in02&~in02)|(in03&~in03)|(in04&~in04)|(in05&~in05)|(in06&~in06)|(in07&~in07)|(in08&~in08)|(in09&~in09)  precision=Full  arith_type=Unsigned  n_bits=8  bin_pt=2  align_bp=on  latency=0  explicit_period=off  period=1  en=off  dbl_ovrd=off  show_param=off
      settings: xl_area=[0, 0, 0, 0, 0, 0, 0]
  expr5 : xbsIndex_r3/Expression  expression=(in03)|(in00&~in00)|(in01&~in01)|(in02&~in02)|(in03&~in03)|(in04&~in04)|(in05&~in05)|(in06&~in06)|(in07&~in07)|(in08&~in08)|(in09&~in09)  precision=Full  arith_type=Unsigned  n_bits=8  bin_pt=2  align_bp=on  latency=0  explicit_period=off  period=1  en=off  dbl_ovrd=off  show_param=off
      settings: xl_area=[0, 0, 0, 0, 0, 0, 0]
  expr6 : xbsIndex_r3/Expression  expression=(in02)|(in00&~in00)|(in01&~in01)|(in02&~in02)|(in03&~in03)|(in04&~in04)|(in05&~in05)|(in06&~in06)|(in07&~in07)|(in08&~in08)|(in09&~in09)  precision=Full  arith_type=Unsigned  n_bits=8  bin_pt=2  align_bp=on  latency=0  explicit_period=off  period=1  en=off  dbl_ovrd=off  show_param=off
      settings: xl_area=[0, 0, 0, 0, 0, 0, 0]
  expr7 : xbsIndex_r3/Expression  expression=(in01)|(in00&~in00)|(in01&~in01)|(in02&~in02)|(in03&~in03)|(in04&~in04)|(in05&~in05)|(in06&~in06)|(in07&~in07)|(in08&~in08)|(in09&~in09)  precision=Full  arith_type=Unsigned  n_bits=8  bin_pt=2  align_bp=on  latency=0  explicit_period=off  period=1  en=off  dbl_ovrd=off  show_param=off
      settings: xl_area=[0, 0, 0, 0, 0, 0, 0]
  expr8 : xbsIndex_r3/Expression  expression=(in00)|(in00&~in00)|(in01&~in01)|(in02&~in02)|(in03&~in03)|(in04&~in04)|(in05&~in05)|(in06&~in06)|(in07&~in07)|(in08&~in08)|(in09&~in09)  precision=Full  arith_type=Unsigned  n_bits=8  bin_pt=2  align_bp=on  latency=0  explicit_period=off  period=1  en=off  dbl_ovrd=off  show_param=off
      settings: xl_area=[0, 0, 0, 0, 0, 0, 0]
  expr9 : xbsIndex_r3/Expression  expression=(~in09)|(in00&~in00)|(in01&~in01)|(in02&~in02)|(in03&~in03)|(in04&~in04)|(in05&~in05)|(in06&~in06)|(in07&~in07)|(in08&~in08)|(in09&~in09)  precision=Full  arith_type=Unsigned  n_bits=8  bin_pt=2  align_bp=on  latency=0  explicit_period=off  period=1  en=off  dbl_ovrd=off  show_param=off
      settings: xl_area=[0, 0, 0, 0, 0, 0, 0]
  dout : Outport
  wires:
  Uncram/10(Out10) -> expr0/1, expr1/1, expr2/1, expr3/1, expr4/1, expr5/1, expr6/1, expr7/1, expr8/1, expr9/1
  Uncram/9(Out9) -> expr0/2, expr1/2, expr2/2, expr3/2, expr4/2, expr5/2, expr6/2, expr7/2, expr8/2, expr9/2
  Uncram/8(Out8) -> expr0/3, expr1/3, expr2/3, expr3/3, expr4/3, expr5/3, expr6/3, expr7/3, expr8/3, expr9/3
  Uncram/7(Out7) -> expr0/4, expr1/4, expr2/4, expr3/4, expr4/4, expr5/4, expr6/4, expr7/4, expr8/4, expr9/4
  Uncram/6(Out6) -> expr0/5, expr1/5, expr2/5, expr3/5, expr4/5, expr5/5, expr6/5, expr7/5, expr8/5, expr9/5
  Uncram/5(Out5) -> expr0/6, expr1/6, expr2/6, expr3/6, expr4/6, expr5/6, expr6/6, expr7/6, expr8/6, expr9/6
  Uncram/4(Out4) -> expr0/7, expr1/7, expr2/7, expr3/7, expr4/7, expr5/7, expr6/7, expr7/7, expr8/7, expr9/7
  Uncram/3(Out3) -> expr0/8, expr1/8, expr2/8, expr3/8, expr4/8, expr5/8, expr6/8, expr7/8, expr8/8, expr9/8
  Uncram/2(Out2) -> expr0/9, expr1/9, expr2/9, expr3/9, expr4/9, expr5/9, expr6/9, expr7/9, expr8/9, expr9/9
  Uncram/1(Out1) -> expr0/10, expr1/10, expr2/10, expr3/10, expr4/10, expr5/10, expr6/10, expr7/10, expr8/10, expr9/10
  expr0/1 -> Concat/10
  expr1/1 -> Concat/9
  expr2/1 -> Concat/8
  expr3/1 -> Concat/7
  expr4/1 -> Concat/6
  expr5/1 -> Concat/5
  expr6/1 -> Concat/4
  expr7/1 -> Concat/3
  expr8/1 -> Concat/2
  expr9/1 -> Concat/1
  din/1 -> Uncram/1(In)
  Concat/1 -> dout/1

== system meat_1024pt_lwip_led/fft/fft_biplex0/biplex_core/fft_stage_1/butterfly/c_to_ri ==
  c : Inport  Port=1  LatchInput=off
  Reinterpret : xbsIndex_r3/Reinterpret  force_arith_type=on  arith_type="Signed  (2's comp)"  force_bin_pt=on  bin_pt=BitWidth - 1  force_valid=on
  Reinterpret1 : xbsIndex_r3/Reinterpret  force_arith_type=on  arith_type="Signed  (2's comp)"  force_bin_pt=on  bin_pt=BitWidth - 1  force_valid=on
  Slice : xbsIndex_r3/Slice  mode=Upper Bit Location + Width  nbits=BitWidth  bit1=0  base1=MSB of Input  bit0=0  base0=LSB of Input  boolean_output=off  explicit_period=off  period=1  dbl_ovrd=off
  Slice1 : xbsIndex_r3/Slice  mode=Lower Bit Location + Width  nbits=BitWidth  bit1=0  base1=MSB of Input  bit0=0  base0=LSB of Input  boolean_output=off  explicit_period=off  period=1  dbl_ovrd=off
  re : Outport
  im : Outport  Port=2
  wires:
  Slice/1 -> Reinterpret/1
  Slice1/1 -> Reinterpret1/1
  Reinterpret/1 -> re/1
  Reinterpret1/1 -> im/1
  c/1 -> Slice/1, Slice1/1

== system meat_1024pt_lwip_led/fft/fft_biplex0/biplex_core/fft_stage_1/butterfly/c_to_ri1 ==
  c : Inport  Port=1  LatchInput=off
  Reinterpret : xbsIndex_r3/Reinterpret  force_arith_type=on  arith_type="Signed  (2's comp)"  force_bin_pt=on  bin_pt=BitWidth - 1  force_valid=on
  Reinterpret1 : xbsIndex_r3/Reinterpret  force_arith_type=on  arith_type="Signed  (2's comp)"  force_bin_pt=on  bin_pt=BitWidth - 1  force_valid=on
  Slice : xbsIndex_r3/Slice  mode=Upper Bit Location + Width  nbits=BitWidth  bit1=0  base1=MSB of Input  bit0=0  base0=LSB of Input  boolean_output=off  explicit_period=off  period=1  dbl_ovrd=off
  Slice1 : xbsIndex_r3/Slice  mode=Lower Bit Location + Width  nbits=BitWidth  bit1=0  base1=MSB of Input  bit0=0  base0=LSB of Input  boolean_output=off  explicit_period=off  period=1  dbl_ovrd=off
  re : Outport
  im : Outport  Port=2
  wires:
  c/1 -> Slice1/1, Slice/1
  Reinterpret1/1 -> im/1
  Reinterpret/1 -> re/1
  Slice1/1 -> Reinterpret1/1
  Slice/1 -> Reinterpret/1

== system meat_1024pt_lwip_led/fft/fft_biplex0/biplex_core/fft_stage_1/butterfly/ri_to_c ==
  re : Inport  Port=1  LatchInput=off
  im : Inport  Port=2  LatchInput=off
  Concat : xbsIndex_r3/Concat  num_inputs=2  explicit_period=off  period=1  dbl_ovrd=off
  Reinterpret : xbsIndex_r3/Reinterpret  force_arith_type=on  arith_type=Unsigned  force_bin_pt=on  bin_pt=0  force_valid=on
  Reinterpret1 : xbsIndex_r3/Reinterpret  force_arith_type=on  arith_type=Unsigned  force_bin_pt=on  bin_pt=0  force_valid=on
  c : Outport
  wires:
  Reinterpret/1 -> Concat/1
  Reinterpret1/1 -> Concat/2
  re/1 -> Reinterpret/1
  Concat/1 -> c/1
  im/1 -> Reinterpret1/1

== system meat_1024pt_lwip_led/fft/fft_biplex0/biplex_core/fft_stage_1/butterfly/ri_to_c1 ==
  re : Inport  Port=1  LatchInput=off
  im : Inport  Port=2  LatchInput=off
  Concat : xbsIndex_r3/Concat  num_inputs=2  explicit_period=off  period=1  dbl_ovrd=off
  Reinterpret : xbsIndex_r3/Reinterpret  force_arith_type=on  arith_type=Unsigned  force_bin_pt=on  bin_pt=0  force_valid=on
  Reinterpret1 : xbsIndex_r3/Reinterpret  force_arith_type=on  arith_type=Unsigned  force_bin_pt=on  bin_pt=0  force_valid=on
  c : Outport
  wires:
  Reinterpret/1 -> Concat/1
  Reinterpret1/1 -> Concat/2
  re/1 -> Reinterpret/1
  Concat/1 -> c/1
  im/1 -> Reinterpret1/1

== system meat_1024pt_lwip_led/fft/fft_biplex0/biplex_core/fft_stage_10/butterfly_direct/twiddle ==
  a : Inport  Port=1  LatchInput=off
  b : Inport  Port=2  LatchInput=off
  sync : Inport  Port=3  LatchInput=off
  twiddle_general_3mult : casper_library/FFTs/Twiddle/twiddle_general_3mult  Coeffs=[exp(-2*pi*1j*(bit_rev(Coeffs, FFTSize-1))/2^FFTSize)]  StepPeriod=0  BitWidth=18  add_latency=3  mult_latency=4  bram_latency=3
  a_re : Outport
  a_im : Outport  Port=2
  bw_re : Outport  Port=3
  bw_im : Outport  Port=4
  sync_out : Outport  Port=5
  wires:
  a/1 -> twiddle_general_3mult/1
  b/1 -> twiddle_general_3mult/2
  sync/1 -> twiddle_general_3mult/3
  twiddle_general_3mult/1 -> a_re/1
  twiddle_general_3mult/2 -> a_im/1
  twiddle_general_3mult/3 -> bw_re/1
  twiddle_general_3mult/4 -> bw_im/1
  twiddle_general_3mult/5 -> sync_out/1

== system meat_1024pt_lwip_led/fft/fft_biplex0/biplex_core/fft_stage_2/butterfly_direct/twiddle ==
  a : Inport  Port=1  LatchInput=off
  b : Inport  Port=2  LatchInput=off
  sync : Inport  Port=3  LatchInput=off
  twiddle_stage_2 : casper_library/FFTs/Twiddle/twiddle_stage_2  FFTSize=10  BitWidth=18  add_latency=3  mult_latency=4  bram_latency=3
  a_re : Outport
  a_im : Outport  Port=2
  bw_re : Outport  Port=3
  bw_im : Outport  Port=4
  sync_out : Outport  Port=5
  wires:
  a/1 -> twiddle_stage_2/1
  b/1 -> twiddle_stage_2/2
  sync/1 -> twiddle_stage_2/3
  twiddle_stage_2/1 -> a_re/1
  twiddle_stage_2/2 -> a_im/1
  twiddle_stage_2/3 -> bw_re/1
  twiddle_stage_2/4 -> bw_im/1
  twiddle_stage_2/5 -> sync_out/1

== system meat_1024pt_lwip_led/fft/fft_biplex0/biplex_core/fft_stage_3/butterfly_direct/twiddle ==
  a : Inport  Port=1  LatchInput=off
  b : Inport  Port=2  LatchInput=off
  sync : Inport  Port=3  LatchInput=off
  twiddle_general_3mult : casper_library/FFTs/Twiddle/twiddle_general_3mult  Coeffs=[exp(-2*pi*1j*(bit_rev(Coeffs, FFTSize-1))/2^FFTSize)]  StepPeriod=7  BitWidth=18  add_latency=3  mult_latency=4  bram_latency=3
  a_re : Outport
  a_im : Outport  Port=2
  bw_re : Outport  Port=3
  bw_im : Outport  Port=4
  sync_out : Outport  Port=5
  wires:
  a/1 -> twiddle_general_3mult/1
  b/1 -> twiddle_general_3mult/2
  sync/1 -> twiddle_general_3mult/3
  twiddle_general_3mult/1 -> a_re/1
  twiddle_general_3mult/2 -> a_im/1
  twiddle_general_3mult/3 -> bw_re/1
  twiddle_general_3mult/4 -> bw_im/1
  twiddle_general_3mult/5 -> sync_out/1

== system meat_1024pt_lwip_led/fft/fft_biplex0/biplex_core/fft_stage_4/butterfly_direct/twiddle ==
  a : Inport  Port=1  LatchInput=off
  b : Inport  Port=2  LatchInput=off
  sync : Inport  Port=3  LatchInput=off
  twiddle_general_3mult : casper_library/FFTs/Twiddle/twiddle_general_3mult  Coeffs=[exp(-2*pi*1j*(bit_rev(Coeffs, FFTSize-1))/2^FFTSize)]  StepPeriod=6  BitWidth=18  add_latency=3  mult_latency=4  bram_latency=3
  a_re : Outport
  a_im : Outport  Port=2
  bw_re : Outport  Port=3
  bw_im : Outport  Port=4
  sync_out : Outport  Port=5
  wires:
  a/1 -> twiddle_general_3mult/1
  b/1 -> twiddle_general_3mult/2
  sync/1 -> twiddle_general_3mult/3
  twiddle_general_3mult/1 -> a_re/1
  twiddle_general_3mult/2 -> a_im/1
  twiddle_general_3mult/3 -> bw_re/1
  twiddle_general_3mult/4 -> bw_im/1
  twiddle_general_3mult/5 -> sync_out/1

== system meat_1024pt_lwip_led/fft/fft_biplex0/biplex_core/fft_stage_5/butterfly_direct/twiddle ==
  a : Inport  Port=1  LatchInput=off
  b : Inport  Port=2  LatchInput=off
  sync : Inport  Port=3  LatchInput=off
  twiddle_general_3mult : casper_library/FFTs/Twiddle/twiddle_general_3mult  Coeffs=[exp(-2*pi*1j*(bit_rev(Coeffs, FFTSize-1))/2^FFTSize)]  StepPeriod=5  BitWidth=18  add_latency=3  mult_latency=4  bram_latency=3
  a_re : Outport
  a_im : Outport  Port=2
  bw_re : Outport  Port=3
  bw_im : Outport  Port=4
  sync_out : Outport  Port=5
  wires:
  a/1 -> twiddle_general_3mult/1
  b/1 -> twiddle_general_3mult/2
  sync/1 -> twiddle_general_3mult/3
  twiddle_general_3mult/1 -> a_re/1
  twiddle_general_3mult/2 -> a_im/1
  twiddle_general_3mult/3 -> bw_re/1
  twiddle_general_3mult/4 -> bw_im/1
  twiddle_general_3mult/5 -> sync_out/1

== system meat_1024pt_lwip_led/fft/fft_biplex0/biplex_core/fft_stage_6/butterfly_direct/twiddle ==
  a : Inport  Port=1  LatchInput=off
  b : Inport  Port=2  LatchInput=off
  sync : Inport  Port=3  LatchInput=off
  twiddle_general_3mult : casper_library/FFTs/Twiddle/twiddle_general_3mult  Coeffs=[exp(-2*pi*1j*(bit_rev(Coeffs, FFTSize-1))/2^FFTSize)]  StepPeriod=4  BitWidth=18  add_latency=3  mult_latency=4  bram_latency=3
  a_re : Outport
  a_im : Outport  Port=2
  bw_re : Outport  Port=3
  bw_im : Outport  Port=4
  sync_out : Outport  Port=5
  wires:
  a/1 -> twiddle_general_3mult/1
  b/1 -> twiddle_general_3mult/2
  sync/1 -> twiddle_general_3mult/3
  twiddle_general_3mult/1 -> a_re/1
  twiddle_general_3mult/2 -> a_im/1
  twiddle_general_3mult/3 -> bw_re/1
  twiddle_general_3mult/4 -> bw_im/1
  twiddle_general_3mult/5 -> sync_out/1

== system meat_1024pt_lwip_led/fft/fft_biplex0/biplex_core/fft_stage_7/butterfly_direct/twiddle ==
  a : Inport  Port=1  LatchInput=off
  b : Inport  Port=2  LatchInput=off
  sync : Inport  Port=3  LatchInput=off
  twiddle_general_3mult : casper_library/FFTs/Twiddle/twiddle_general_3mult  Coeffs=[exp(-2*pi*1j*(bit_rev(Coeffs, FFTSize-1))/2^FFTSize)]  StepPeriod=3  BitWidth=18  add_latency=3  mult_latency=4  bram_latency=3
  a_re : Outport
  a_im : Outport  Port=2
  bw_re : Outport  Port=3
  bw_im : Outport  Port=4
  sync_out : Outport  Port=5
  wires:
  a/1 -> twiddle_general_3mult/1
  b/1 -> twiddle_general_3mult/2
  sync/1 -> twiddle_general_3mult/3
  twiddle_general_3mult/1 -> a_re/1
  twiddle_general_3mult/2 -> a_im/1
  twiddle_general_3mult/3 -> bw_re/1
  twiddle_general_3mult/4 -> bw_im/1
  twiddle_general_3mult/5 -> sync_out/1

== system meat_1024pt_lwip_led/fft/fft_biplex0/biplex_core/fft_stage_8/butterfly_direct/twiddle ==
  a : Inport  Port=1  LatchInput=off
  b : Inport  Port=2  LatchInput=off
  sync : Inport  Port=3  LatchInput=off
  twiddle_general_3mult : casper_library/FFTs/Twiddle/twiddle_general_3mult  Coeffs=[exp(-2*pi*1j*(bit_rev(Coeffs, FFTSize-1))/2^FFTSize)]  StepPeriod=2  BitWidth=18  add_latency=3  mult_latency=4  bram_latency=3
  a_re : Outport
  a_im : Outport  Port=2
  bw_re : Outport  Port=3
  bw_im : Outport  Port=4
  sync_out : Outport  Port=5
  wires:
  a/1 -> twiddle_general_3mult/1
  b/1 -> twiddle_general_3mult/2
  sync/1 -> twiddle_general_3mult/3
  twiddle_general_3mult/1 -> a_re/1
  twiddle_general_3mult/2 -> a_im/1
  twiddle_general_3mult/3 -> bw_re/1
  twiddle_general_3mult/4 -> bw_im/1
  twiddle_general_3mult/5 -> sync_out/1

== system meat_1024pt_lwip_led/fft/fft_biplex0/biplex_core/fft_stage_9/butterfly_direct/twiddle ==
  a : Inport  Port=1  LatchInput=off
  b : Inport  Port=2  LatchInput=off
  sync : Inport  Port=3  LatchInput=off
  twiddle_general_3mult : casper_library/FFTs/Twiddle/twiddle_general_3mult  Coeffs=[exp(-2*pi*1j*(bit_rev(Coeffs, FFTSize-1))/2^FFTSize)]  StepPeriod=1  BitWidth=18  add_latency=3  mult_latency=4  bram_latency=3
  a_re : Outport
  a_im : Outport  Port=2
  bw_re : Outport  Port=3
  bw_im : Outport  Port=4
  sync_out : Outport  Port=5
  wires:
  a/1 -> twiddle_general_3mult/1
  b/1 -> twiddle_general_3mult/2
  sync/1 -> twiddle_general_3mult/3
  twiddle_general_3mult/1 -> a_re/1
  twiddle_general_3mult/2 -> a_im/1
  twiddle_general_3mult/3 -> bw_re/1
  twiddle_general_3mult/4 -> bw_im/1
  twiddle_general_3mult/5 -> sync_out/1

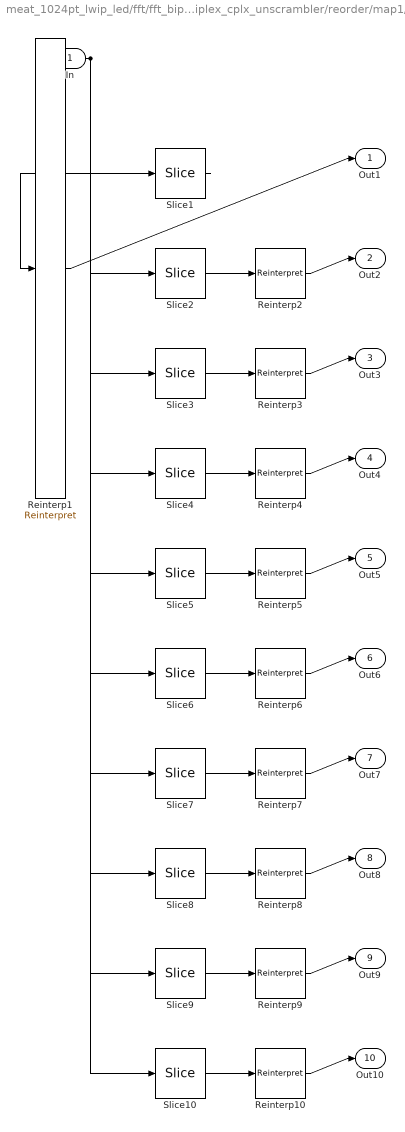
== system meat_1024pt_lwip_led/fft/fft_biplex0/biplex_cplx_unscrambler/reorder/map1/Uncram ==
  In : Inport  Port=1  LatchInput=off
  Reinterp{1..10} (10 alike) : xbsIndex_r3/Reinterpret  force_arith_type=on  arith_type=Unsigned  force_bin_pt=on  bin_pt=0  force_valid=on
  Slice1 : xbsIndex_r3/Slice  mode=Upper Bit Location + Width  nbits=1  bit1=0  base1=MSB of Input  bit0=0  base0=LSB of Input  boolean_output=off  explicit_period=off  period=1  dbl_ovrd=off
  Slice10 : xbsIndex_r3/Slice  mode=Upper Bit Location + Width  nbits=1  bit1=-9  base1=MSB of Input  bit0=0  base0=LSB of Input  boolean_output=off  explicit_period=off  period=1  dbl_ovrd=off
  Slice2 : xbsIndex_r3/Slice  mode=Upper Bit Location + Width  nbits=1  bit1=-1  base1=MSB of Input  bit0=0  base0=LSB of Input  boolean_output=off  explicit_period=off  period=1  dbl_ovrd=off
  Slice3 : xbsIndex_r3/Slice  mode=Upper Bit Location + Width  nbits=1  bit1=-2  base1=MSB of Input  bit0=0  base0=LSB of Input  boolean_output=off  explicit_period=off  period=1  dbl_ovrd=off
  Slice4 : xbsIndex_r3/Slice  mode=Upper Bit Location + Width  nbits=1  bit1=-3  base1=MSB of Input  bit0=0  base0=LSB of Input  boolean_output=off  explicit_period=off  period=1  dbl_ovrd=off
  Slice5 : xbsIndex_r3/Slice  mode=Upper Bit Location + Width  nbits=1  bit1=-4  base1=MSB of Input  bit0=0  base0=LSB of Input  boolean_output=off  explicit_period=off  period=1  dbl_ovrd=off
  Slice6 : xbsIndex_r3/Slice  mode=Upper Bit Location + Width  nbits=1  bit1=-5  base1=MSB of Input  bit0=0  base0=LSB of Input  boolean_output=off  explicit_period=off  period=1  dbl_ovrd=off
  Slice7 : xbsIndex_r3/Slice  mode=Upper Bit Location + Width  nbits=1  bit1=-6  base1=MSB of Input  bit0=0  base0=LSB of Input  boolean_output=off  explicit_period=off  period=1  dbl_ovrd=off
  Slice8 : xbsIndex_r3/Slice  mode=Upper Bit Location + Width  nbits=1  bit1=-7  base1=MSB of Input  bit0=0  base0=LSB of Input  boolean_output=off  explicit_period=off  period=1  dbl_ovrd=off
  Slice9 : xbsIndex_r3/Slice  mode=Upper Bit Location + Width  nbits=1  bit1=-8  base1=MSB of Input  bit0=0  base0=LSB of Input  boolean_output=off  explicit_period=off  period=1  dbl_ovrd=off
  Out1 : Outport
  Out2 : Outport  Port=2
  Out3 : Outport  Port=3
  Out4 : Outport  Port=4
  Out5 : Outport  Port=5
  Out6 : Outport  Port=6
  Out7 : Outport  Port=7
  Out8 : Outport  Port=8
  Out9 : Outport  Port=9
  Out10 : Outport  Port=10
  wires:
  In/1 -> Slice1/1, Slice2/1, Slice3/1, Slice4/1, Slice5/1, Slice6/1, Slice7/1, Slice8/1, Slice9/1, Slice10/1
  Slice1/1 -> Reinterp1/1
  Reinterp1/1 -> Out1/1
  Slice2/1 -> Reinterp2/1
  Reinterp2/1 -> Out2/1
  Slice3/1 -> Reinterp3/1
  Reinterp3/1 -> Out3/1
  Slice4/1 -> Reinterp4/1
  Reinterp4/1 -> Out4/1
  Slice5/1 -> Reinterp5/1
  Reinterp5/1 -> Out5/1
  Slice6/1 -> Reinterp6/1
  Reinterp6/1 -> Out6/1
  Slice7/1 -> Reinterp7/1
  Reinterp7/1 -> Out7/1
  Slice8/1 -> Reinterp8/1
  Reinterp8/1 -> Out8/1
  Slice9/1 -> Reinterp9/1
  Reinterp9/1 -> Out9/1
  Slice10/1 -> Reinterp10/1
  Reinterp10/1 -> Out10/1

== system meat_1024pt_lwip_led/fft/fft_biplex0/biplex_cplx_unscrambler/reorder1/map1/Uncram ==
  In : Inport  Port=1  LatchInput=off
  Reinterp{1..10} (10 alike) : xbsIndex_r3/Reinterpret  force_arith_type=on  arith_type=Unsigned  force_bin_pt=on  bin_pt=0  force_valid=on
  Slice1 : xbsIndex_r3/Slice  mode=Upper Bit Location + Width  nbits=1  bit1=0  base1=MSB of Input  bit0=0  base0=LSB of Input  boolean_output=off  explicit_period=off  period=1  dbl_ovrd=off
  Slice10 : xbsIndex_r3/Slice  mode=Upper Bit Location + Width  nbits=1  bit1=-9  base1=MSB of Input  bit0=0  base0=LSB of Input  boolean_output=off  explicit_period=off  period=1  dbl_ovrd=off
  Slice2 : xbsIndex_r3/Slice  mode=Upper Bit Location + Width  nbits=1  bit1=-1  base1=MSB of Input  bit0=0  base0=LSB of Input  boolean_output=off  explicit_period=off  period=1  dbl_ovrd=off
  Slice3 : xbsIndex_r3/Slice  mode=Upper Bit Location + Width  nbits=1  bit1=-2  base1=MSB of Input  bit0=0  base0=LSB of Input  boolean_output=off  explicit_period=off  period=1  dbl_ovrd=off
  Slice4 : xbsIndex_r3/Slice  mode=Upper Bit Location + Width  nbits=1  bit1=-3  base1=MSB of Input  bit0=0  base0=LSB of Input  boolean_output=off  explicit_period=off  period=1  dbl_ovrd=off
  Slice5 : xbsIndex_r3/Slice  mode=Upper Bit Location + Width  nbits=1  bit1=-4  base1=MSB of Input  bit0=0  base0=LSB of Input  boolean_output=off  explicit_period=off  period=1  dbl_ovrd=off
  Slice6 : xbsIndex_r3/Slice  mode=Upper Bit Location + Width  nbits=1  bit1=-5  base1=MSB of Input  bit0=0  base0=LSB of Input  boolean_output=off  explicit_period=off  period=1  dbl_ovrd=off
  Slice7 : xbsIndex_r3/Slice  mode=Upper Bit Location + Width  nbits=1  bit1=-6  base1=MSB of Input  bit0=0  base0=LSB of Input  boolean_output=off  explicit_period=off  period=1  dbl_ovrd=off
  Slice8 : xbsIndex_r3/Slice  mode=Upper Bit Location + Width  nbits=1  bit1=-7  base1=MSB of Input  bit0=0  base0=LSB of Input  boolean_output=off  explicit_period=off  period=1  dbl_ovrd=off
  Slice9 : xbsIndex_r3/Slice  mode=Upper Bit Location + Width  nbits=1  bit1=-8  base1=MSB of Input  bit0=0  base0=LSB of Input  boolean_output=off  explicit_period=off  period=1  dbl_ovrd=off
  Out1 : Outport
  Out2 : Outport  Port=2
  Out3 : Outport  Port=3
  Out4 : Outport  Port=4
  Out5 : Outport  Port=5
  Out6 : Outport  Port=6
  Out7 : Outport  Port=7
  Out8 : Outport  Port=8
  Out9 : Outport  Port=9
  Out10 : Outport  Port=10
  wires:
  In/1 -> Slice1/1, Slice2/1, Slice3/1, Slice4/1, Slice5/1, Slice6/1, Slice7/1, Slice8/1, Slice9/1, Slice10/1
  Slice1/1 -> Reinterp1/1
  Reinterp1/1 -> Out1/1
  Slice2/1 -> Reinterp2/1
  Reinterp2/1 -> Out2/1
  Slice3/1 -> Reinterp3/1
  Reinterp3/1 -> Out3/1
  Slice4/1 -> Reinterp4/1
  Reinterp4/1 -> Out4/1
  Slice5/1 -> Reinterp5/1
  Reinterp5/1 -> Out5/1
  Slice6/1 -> Reinterp6/1
  Reinterp6/1 -> Out6/1
  Slice7/1 -> Reinterp7/1
  Reinterp7/1 -> Out7/1
  Slice8/1 -> Reinterp8/1
  Reinterp8/1 -> Out8/1
  Slice9/1 -> Reinterp9/1
  Reinterp9/1 -> Out9/1
  Slice10/1 -> Reinterp10/1
  Reinterp10/1 -> Out10/1
